simulink model "p82015"  (R2015a)
settings: Solver=ode45  SolverMode=SingleTasking  StartTime=0.0  StopTime=20  RelTol=1e-3
libraries: fl_lib x11, nesl_utility x6
settings Model: CovMetricSettings=dwe  CovHtmlReporting=off  covSaveCumulativeToWorkspaceVar=off  CovSaveSingleToWorkspaceVar=off  CovExternalEMLEnable=on  Creator=Jesus  LastModifiedBy=linux
settings DataIOCC: LimitDataPoints=off  SaveFormat=Dataset
settings DebuggingCC: SFUnexpectedBacktrackingDiag=error  SFNoUnconditionalDefaultTransitionDiag=error
settings HardwareCC: ProdBitPerPointer=64  ProdLargestAtomicFloat=Float  ProdIntDivRoundTo=Zero  ProdEndianess=LittleEndian  ProdHWDeviceType=Specified
settings ModelReferenceCC: PropagateSignalLabelsOutOfModel=on
settings GRTTargetCC: TargetLangStandard=C99 (ISO)  GeneratePreprocessorConditionals=Use local settings

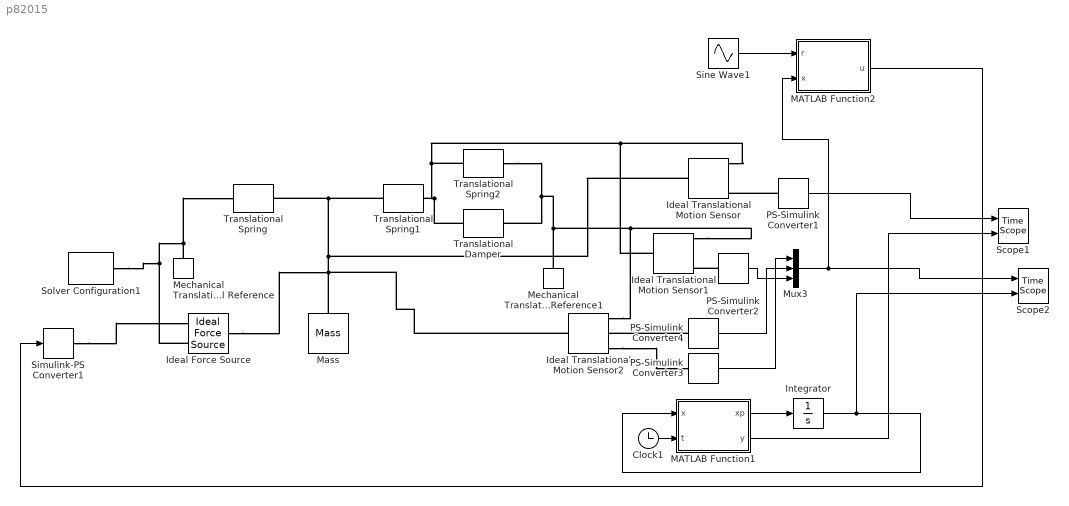
== system p82015 ==
  Clock1 : Clock
  Ideal Force Source : fl_lib/Mechanical/Mechanical Sources/Ideal Force Source
  Ideal Translational Motion Sensor : fl_lib/Mechanical/Mechanical Sensors/Ideal Translational Motion Sensor  offset=0 m
  Ideal Translational Motion Sensor1 : fl_lib/Mechanical/Mechanical Sensors/Ideal Translational Motion Sensor  offset=0 m
  Ideal Translational Motion Sensor2 : fl_lib/Mechanical/Mechanical Sensors/Ideal Translational Motion Sensor  offset=0 m
  Integrator : Integrator  InitialCondition=[0 0 0]
  MATLAB Function1 : MATLAB Function  TreatAsAtomicUnit=on
  MATLAB Function2 : MATLAB Function  TreatAsAtomicUnit=on
  Mass : fl_lib/Mechanical/Translational Elements/Mass  mass=10 kg  v_specify=off  v_priority=High  v=0 m/s  f_specify=off  f_priority=High  f=0 N
  Mechanical Translational Reference : fl_lib/Mechanical/Translational Elements/Mechanical Translational Reference
  Mechanical Translational Reference1 : fl_lib/Mechanical/Translational Elements/Mechanical Translational Reference
  Mux3 : Mux  Inputs=3
  PS-Simulink Converter{1..4} (4 alike) : nesl_utility/PS-Simulink Converter  PhysicalDomain=network_engine_domain  SubClassName=ps_output  LeftPortType=input  RightPortType=output  PseudoPeriodic=off  Frequencies=[]  Unit=1  AffineConversion=off
  Scope1 : TimeScope  NumInputPorts=2
  Scope2 : TimeScope  NumInputPorts=2
  Simulink-PS Converter1 : nesl_utility/Simulink-PS Converter  PhysicalDomain=network_engine_domain  SubClassName=ps_input  LeftPortType=input  RightPortType=output  PseudoPeriodic=off  Frequencies=[]  NoiseDistribution=none  NoiseParameters=[]  Unit=1  AffineConversion=off  InputFiltering=off  SimscapeFilterOrder=1  InputFilterTimeConstant=0.001  UdotUserProvided=0
  Sine Wave1 : Sin  SampleTime=0
  Solver Configuration1 : nesl_utility/Solver Configuration  PhysicalDomain=network_engine_domain  SubClassName=solver  LeftPortType=input  RightPortType=generic  Accelerate=off  Tones=[]  Harmonics=[]  SimulateNoise=off  Profile=off  UseLocalSampling=off  EnableSwitchedLinearOptims=on  FrequencyDomain=off  UseCCode=off  RelTol=0.001  AbsTol=1e-06  MinStep=1e-09  ToWorkspace=off  RevertToSquareIcSolve=off  NumHomotopyIterations=100  DoDC=off  ResidualTolerance=1e-09  UseLocalSolver=off  LocalSolverChoice=NE_BACKWARD_EULER_ADVANCER  LocalSolverSampleTime=0.001  DoFixedCost=off  MaxNonlinIter=3  MaxModeIter=2  LinearAlgebra=Sparse  DelaysMemoryBudget=1024  AutomaticFiltering=on  FilteringTimeConstant=0.001
  Translational Damper : fl_lib/Mechanical/Translational Elements/Translational Damper  D=.5 N/(m/s)  v_specify=off  v_priority=High  v=0 m/s  f_specify=off  f_priority=High  f=0 N
  Translational Spring : fl_lib/Mechanical/Translational Elements/Translational Spring  spr_rate=2 N/m  v_specify=off  v_priority=High  v=0 m/s  f_specify=off  f_priority=High  f=0 N  x_specify=off  x_priority=High  x=0 m
  Translational Spring1 : fl_lib/Mechanical/Translational Elements/Translational Spring  spr_rate=1 N/m  v_specify=off  v_priority=High  v=0 m/s  f_specify=off  f_priority=High  f=0 N  x_specify=off  x_priority=High  x=0 m
  Translational Spring2 : fl_lib/Mechanical/Translational Elements/Translational Spring  spr_rate=.5 N/m  v_specify=off  v_priority=High  v=0 m/s  f_specify=off  f_priority=High  f=0 N  x_specify=off  x_priority=High  x=0 m
  wires:
  PS-Simulink Converter1/1 -> Scope1/1
  MATLAB Function1/1(xp) -> Integrator/1
  Clock1/1 -> MATLAB Function1/2(t)
  MATLAB Function1/2(y) -> Scope1/2
  PS-Simulink Converter3/1 -> Mux3/1
  PS-Simulink Converter4/1 -> Mux3/2
  PS-Simulink Converter2/1 -> Mux3/3
  Mux3/1 -> Scope2/1, MATLAB Function2/2(x)
  Sine Wave1/1 -> MATLAB Function2/1(r)
  MATLAB Function2/1(u) -> Simulink-PS Converter1/1
  Integrator/1 -> Scope2/2, MATLAB Function1/1(x)
  connections:
  Mass/LConn1 -- Ideal Translational Motion Sensor2/LConn1 -- Ideal Force Source/LConn1 -- Translational Spring1/LConn1 -- Translational Spring/RConn1 -- Ideal Translational Motion Sensor/LConn1
  Mechanical Translational Reference/LConn1 -- Solver Configuration1/RConn1 -- Ideal Force Source/RConn2 -- Translational Spring/LConn1
  Translational Spring2/LConn1 -- Ideal Translational Motion Sensor/RConn1 -- Ideal Translational Motion Sensor1/LConn1 -- Translational Damper/LConn1 -- Translational Spring1/RConn1
  Translational Spring2/RConn1 -- Ideal Translational Motion Sensor2/RConn1 -- Ideal Translational Motion Sensor1/RConn1 -- Mechanical Translational Reference1/LConn1 -- Translational Damper/RConn1
  PS-Simulink Converter1/LConn1 -- Ideal Translational Motion Sensor/RConn3
  PS-Simulink Converter2/LConn1 -- Ideal Translational Motion Sensor1/RConn3
  Ideal Translational Motion Sensor2/RConn3 -- PS-Simulink Converter3/LConn1
  PS-Simulink Converter4/LConn1 -- Ideal Translational Motion Sensor2/RConn2
  Simulink-PS Converter1/RConn1 -- Ideal Force Source/RConn1

== matlab function p82015/MATLAB Function1 ==
  data: xp output; x input; y output; t input
function [xp,y] = fcn(x,t)
k1=2;
k2=1;
k3=.5;
b1=.5;
m1=10;
K=[87.0000   60.0000    1.0000];
u=sin(t)-K*x;
A=[0,1,0;-(k1/m1)-(k2/m1),0,k2/m1;k2/b1,0,(-k2/b1)-(k3/b1)];
B=[0,1/m1,0]';
C=[1,0,-1];
xp=A*x+B*u;
x12=[x(1),x(3)]
y=C*x;

== matlab function p82015/MATLAB Function2 ==
  data: r input; u output; x input
function u  = fcn(r,x)
K=[87.0000   60.0000    1.0000];
u=r-K*x;
